simulink model "IEEE9_case"  (R2024b)
settings: Solver=FixedStepAuto  StartTime=0  StopTime=5  FixedStep=1e-7  RelTol=1e-3
values from neighbouring files (symbols this model uses):
  SG_D_1_D = 0.01056    [IEEE9_case_parameters.m]    (also in case1_parameters.m; case2_parameters.m; case3_parameters.m; case4_parameters.m)
  SG_D_1_EnableSaturation = 0    [IEEE9_case_parameters.m]    (also in case1_parameters.m; case2_parameters.m; case3_parameters.m; case4_parameters.m)
  SG_D_1_f0 = 60    [IEEE9_case_parameters.m]    (also in case1_parameters.m; case2_parameters.m; case3_parameters.m; case4_parameters.m)
  SG_D_1_H = 7.5    [IEEE9_case_parameters.m]    (also in case1_parameters.m; case2_parameters.m; case3_parameters.m; case4_parameters.m)
  SG_D_1_K_A = 20    [IEEE9_case_parameters.m]    (also in case1_parameters.m; case2_parameters.m; case3_parameters.m; case4_parameters.m)
  SG_D_1_K_E = 1.000000e+1    (= 10)    [IEEE9_case_parameters.m]    (also in case1_parameters.m; case2_parameters.m; case3_parameters.m; case4_parameters.m)
  SG_D_1_K_F = 2.363    [IEEE9_case_parameters.m]    (also in case1_parameters.m; case2_parameters.m; case3_parameters.m; case4_parameters.m)
  SG_D_1_K_s = 0.5    [IEEE9_case_parameters.m]    (also in case1_parameters.m = 5; case2_parameters.m = 5; case3_parameters.m = 5; case4_parameters.m = 5)
  SG_D_1_R_a = 0.001088    [IEEE9_case_parameters.m]    (also in case1_parameters.m; case2_parameters.m; case3_parameters.m; case4_parameters.m)
  SG_D_1_S_A = 1    [IEEE9_case_parameters.m]    (also in case1_parameters.m; case2_parameters.m; case3_parameters.m; case4_parameters.m)
  SG_D_1_S_B = 0.103    [IEEE9_case_parameters.m]    (also in case1_parameters.m; case2_parameters.m; case3_parameters.m; case4_parameters.m)
  SG_D_1_S_N = 10.659857    [IEEE9_case_parameters.m]    (also in case1_parameters.m; case2_parameters.m; case3_parameters.m; case4_parameters.m)
  SG_D_1_SpeedPara = 200    [IEEE9_case_parameters.m]    (also in case1_parameters.m; case2_parameters.m; case3_parameters.m; case4_parameters.m)
  SG_D_1_T_0 = 0.720173    [IEEE9_case_parameters.m]    (also in case1_parameters.m = 0.755522; case2_parameters.m = 0.808931; case3_parameters.m = 0.869402; case4_parameters.m = 0.729316)
  SG_D_1_T_1 = 0.3    [IEEE9_case_parameters.m]    (also in case1_parameters.m; case2_parameters.m; case3_parameters.m; case4_parameters.m)
  SG_D_1_T_2 = 0.05    [IEEE9_case_parameters.m]    (also in case1_parameters.m; case2_parameters.m; case3_parameters.m; case4_parameters.m)
  SG_D_1_T_3 = 0.02    [IEEE9_case_parameters.m]    (also in case1_parameters.m; case2_parameters.m; case3_parameters.m; case4_parameters.m)
  SG_D_1_T_4 = 0.005    [IEEE9_case_parameters.m]    (also in case1_parameters.m; case2_parameters.m; case3_parameters.m; case4_parameters.m)
  SG_D_1_T_A = 0.02    [IEEE9_case_parameters.m]    (also in case1_parameters.m; case2_parameters.m; case3_parameters.m; case4_parameters.m)
  SG_D_1_T_dd = 8.000000e+0    (= 8)    [IEEE9_case_parameters.m]    (also in case1_parameters.m; case2_parameters.m; case3_parameters.m; case4_parameters.m)
  SG_D_1_T_ddd = 0.04    [IEEE9_case_parameters.m]    (also in case1_parameters.m; case2_parameters.m; case3_parameters.m; case4_parameters.m)
  SG_D_1_T_E = 0.314    [IEEE9_case_parameters.m]    (also in case1_parameters.m; case2_parameters.m; case3_parameters.m; case4_parameters.m)
  SG_D_1_T_F = 0.35    [IEEE9_case_parameters.m]    (also in case1_parameters.m; case2_parameters.m; case3_parameters.m; case4_parameters.m)
  SG_D_1_T_qd = 0.8    [IEEE9_case_parameters.m]    (also in case1_parameters.m; case2_parameters.m; case3_parameters.m; case4_parameters.m)
  SG_D_1_T_qdd = 0.02    [IEEE9_case_parameters.m]    (also in case1_parameters.m; case2_parameters.m; case3_parameters.m; case4_parameters.m)
  SG_D_1_T_speed = 0.1    [IEEE9_case_parameters.m]    (also in case1_parameters.m = 200; case2_parameters.m = 200; case3_parameters.m = 200; case4_parameters.m = 200)
  SG_D_1_T_w = 0.5    [IEEE9_case_parameters.m]    (also in case1_parameters.m; case2_parameters.m; case3_parameters.m; case4_parameters.m)
  SG_D_1_V_ref = 1.990276    [IEEE9_case_parameters.m]    (also in case1_parameters.m = 2.042296; case2_parameters.m = 2.051388; case3_parameters.m = 2.089584; case4_parameters.m = 2.01845)
  SG_D_1_w_ref = 376.991118    [IEEE9_case_parameters.m]    (also in case1_parameters.m; case2_parameters.m; case3_parameters.m; case4_parameters.m)
  SG_D_1_wb = 6.000000e+1    (= 60)    [IEEE9_case_parameters.m]    (also in case1_parameters.m; case2_parameters.m; case3_parameters.m; case4_parameters.m)
  SG_D_1_x_d = 1.9    [IEEE9_case_parameters.m]    (also in case1_parameters.m; case2_parameters.m; case3_parameters.m; case4_parameters.m)
  SG_D_1_x_dd = 0.302    [IEEE9_case_parameters.m]    (also in case1_parameters.m; case2_parameters.m; case3_parameters.m; case4_parameters.m)
  SG_D_1_x_ddd = 0.204    [IEEE9_case_parameters.m]    (also in case1_parameters.m; case2_parameters.m; case3_parameters.m; case4_parameters.m)
  SG_D_1_x_l = 0.05    [IEEE9_case_parameters.m]    (also in case1_parameters.m; case2_parameters.m; case3_parameters.m; case4_parameters.m)
  SG_D_1_x_q = 1.3    [IEEE9_case_parameters.m]    (also in case1_parameters.m; case2_parameters.m; case3_parameters.m; case4_parameters.m)
  SG_D_1_x_qd = 0.5    [IEEE9_case_parameters.m]    (also in case1_parameters.m; case2_parameters.m; case3_parameters.m; case4_parameters.m)
  SG_D_1_x_qdd = 0.3    [IEEE9_case_parameters.m]    (also in case1_parameters.m; case2_parameters.m; case3_parameters.m; case4_parameters.m)
  SG_D_2_D = 0.02    [IEEE9_case_parameters.m]    (also in case1_parameters.m; case2_parameters.m; case3_parameters.m; case4_parameters.m)
  SG_D_2_EnableSaturation = 0    [IEEE9_case_parameters.m]    (also in case1_parameters.m; case2_parameters.m; case3_parameters.m; case4_parameters.m)
  SG_D_2_f0 = 60    [IEEE9_case_parameters.m]    (also in case1_parameters.m; case2_parameters.m; case3_parameters.m; case4_parameters.m)
  SG_D_2_H = 8.000000e+0    (= 8)    [IEEE9_case_parameters.m]    (also in case1_parameters.m; case2_parameters.m; case3_parameters.m; case4_parameters.m)
  SG_D_2_K_A = 20    [IEEE9_case_parameters.m]    (also in case1_parameters.m; case2_parameters.m; case3_parameters.m; case4_parameters.m)
  SG_D_2_K_E = 1.000000e+1    (= 10)    [IEEE9_case_parameters.m]    (also in case1_parameters.m; case2_parameters.m; case3_parameters.m; case4_parameters.m)
  SG_D_2_K_F = 2.363    [IEEE9_case_parameters.m]    (also in case1_parameters.m; case2_parameters.m; case3_parameters.m; case4_parameters.m)
  SG_D_2_K_s = 0.5    [IEEE9_case_parameters.m]    (also in case1_parameters.m = 4; case2_parameters.m = 4; case3_parameters.m = 4; case4_parameters.m = 4)
  SG_D_2_R_a = 0.001088    [IEEE9_case_parameters.m]    (also in case1_parameters.m; case2_parameters.m; case3_parameters.m; case4_parameters.m)
  SG_D_2_S_A = 1    [IEEE9_case_parameters.m]    (also in case1_parameters.m; case2_parameters.m; case3_parameters.m; case4_parameters.m)
  SG_D_2_S_B = 0.103    [IEEE9_case_parameters.m]    (also in case1_parameters.m; case2_parameters.m; case3_parameters.m; case4_parameters.m)
  SG_D_2_S_N = 10.659857    [IEEE9_case_parameters.m]    (also in case1_parameters.m; case2_parameters.m; case3_parameters.m; case4_parameters.m)
  SG_D_2_SpeedPara = 200    [IEEE9_case_parameters.m]    (also in case1_parameters.m; case2_parameters.m; case3_parameters.m; case4_parameters.m)
  SG_D_2_T_0 = 1.632913    [IEEE9_case_parameters.m]    (also in case1_parameters.m = 1.632925; case2_parameters.m = 1.632915; case3_parameters.m = 1.632914; case4_parameters.m = 1.632927)
  SG_D_2_T_1 = 0.2    [IEEE9_case_parameters.m]    (also in case1_parameters.m; case2_parameters.m; case3_parameters.m; case4_parameters.m)
  SG_D_2_T_2 = 0.05    [IEEE9_case_parameters.m]    (also in case1_parameters.m; case2_parameters.m; case3_parameters.m; case4_parameters.m)
  SG_D_2_T_3 = 0.02    [IEEE9_case_parameters.m]    (also in case1_parameters.m; case2_parameters.m; case3_parameters.m; case4_parameters.m)
  SG_D_2_T_4 = 0.005    [IEEE9_case_parameters.m]    (also in case1_parameters.m; case2_parameters.m; case3_parameters.m; case4_parameters.m)
  SG_D_2_T_A = 0.02    [IEEE9_case_parameters.m]    (also in case1_parameters.m; case2_parameters.m; case3_parameters.m; case4_parameters.m)
  SG_D_2_T_dd = 7.9    [IEEE9_case_parameters.m]    (also in case1_parameters.m; case2_parameters.m; case3_parameters.m; case4_parameters.m)
  SG_D_2_T_ddd = 0.04    [IEEE9_case_parameters.m]    (also in case1_parameters.m; case2_parameters.m; case3_parameters.m; case4_parameters.m)
  SG_D_2_T_E = 0.314    [IEEE9_case_parameters.m]    (also in case1_parameters.m; case2_parameters.m; case3_parameters.m; case4_parameters.m)
  SG_D_2_T_F = 0.35    [IEEE9_case_parameters.m]    (also in case1_parameters.m; case2_parameters.m; case3_parameters.m; case4_parameters.m)
  SG_D_2_T_qd = 0.8    [IEEE9_case_parameters.m]    (also in case1_parameters.m; case2_parameters.m; case3_parameters.m; case4_parameters.m)
  SG_D_2_T_qdd = 0.015    [IEEE9_case_parameters.m]    (also in case1_parameters.m; case2_parameters.m; case3_parameters.m; case4_parameters.m)
  SG_D_2_T_speed = 0.1    [IEEE9_case_parameters.m]    (also in case1_parameters.m = 150; case2_parameters.m = 150; case3_parameters.m = 150; case4_parameters.m = 150)
  SG_D_2_T_w = 0.35    [IEEE9_case_parameters.m]    (also in case1_parameters.m; case2_parameters.m; case3_parameters.m; case4_parameters.m)
  SG_D_2_V_ref = 2.58547    [IEEE9_case_parameters.m]    (also in case1_parameters.m = 2.597896; case2_parameters.m = 2.587136; case3_parameters.m = 2.586042; case4_parameters.m = 2.599679)
  SG_D_2_w_ref = 376.991118    [IEEE9_case_parameters.m]    (also in case1_parameters.m; case2_parameters.m; case3_parameters.m; case4_parameters.m)
  SG_D_2_wb = 6.000000e+1    (= 60)    [IEEE9_case_parameters.m]    (also in case1_parameters.m; case2_parameters.m; case3_parameters.m; case4_parameters.m)
  SG_D_2_x_d = 1.8    [IEEE9_case_parameters.m]    (also in case1_parameters.m; case2_parameters.m; case3_parameters.m; case4_parameters.m)
  SG_D_2_x_dd = 0.302    [IEEE9_case_parameters.m]    (also in case1_parameters.m; case2_parameters.m; case3_parameters.m; case4_parameters.m)
  SG_D_2_x_ddd = 0.204    [IEEE9_case_parameters.m]    (also in case1_parameters.m; case2_parameters.m; case3_parameters.m; case4_parameters.m)
  SG_D_2_x_l = 0.05    [IEEE9_case_parameters.m]    (also in case1_parameters.m; case2_parameters.m; case3_parameters.m; case4_parameters.m)
  SG_D_2_x_q = 1.25    [IEEE9_case_parameters.m]    (also in case1_parameters.m; case2_parameters.m; case3_parameters.m; case4_parameters.m)
  SG_D_2_x_qd = 0.5    [IEEE9_case_parameters.m]    (also in case1_parameters.m; case2_parameters.m; case3_parameters.m; case4_parameters.m)
  SG_D_2_x_qdd = 0.3    [IEEE9_case_parameters.m]    (also in case1_parameters.m; case2_parameters.m; case3_parameters.m; case4_parameters.m)
  SG_D_3_D = 0.02    [IEEE9_case_parameters.m]    (also in case1_parameters.m; case2_parameters.m; case3_parameters.m; case4_parameters.m)
  SG_D_3_EnableSaturation = 0    [IEEE9_case_parameters.m]    (also in case1_parameters.m; case2_parameters.m; case3_parameters.m; case4_parameters.m)
  SG_D_3_f0 = 60    [IEEE9_case_parameters.m]    (also in case1_parameters.m; case2_parameters.m; case3_parameters.m; case4_parameters.m)
  SG_D_3_H = 7.7    [IEEE9_case_parameters.m]    (also in case1_parameters.m; case2_parameters.m; case3_parameters.m; case4_parameters.m)
  SG_D_3_K_A = 20    [IEEE9_case_parameters.m]    (also in case1_parameters.m; case2_parameters.m; case3_parameters.m; case4_parameters.m)
  SG_D_3_K_E = 1.000000e+1    (= 10)    [IEEE9_case_parameters.m]    (also in case1_parameters.m; case2_parameters.m; case3_parameters.m; case4_parameters.m)
  SG_D_3_K_F = 2.363    [IEEE9_case_parameters.m]    (also in case1_parameters.m; case2_parameters.m; case3_parameters.m; case4_parameters.m)
  SG_D_3_K_s = 0.2    [IEEE9_case_parameters.m]    (also in case1_parameters.m = 2; case2_parameters.m = 2; case3_parameters.m = 2; case4_parameters.m = 2)
  SG_D_3_R_a = 0.001088    [IEEE9_case_parameters.m]    (also in case1_parameters.m; case2_parameters.m; case3_parameters.m; case4_parameters.m)
  SG_D_3_S_A = 1    [IEEE9_case_parameters.m]    (also in case1_parameters.m; case2_parameters.m; case3_parameters.m; case4_parameters.m)
  SG_D_3_S_B = 0.103    [IEEE9_case_parameters.m]    (also in case1_parameters.m; case2_parameters.m; case3_parameters.m; case4_parameters.m)
  SG_D_3_S_N = 10.659857    [IEEE9_case_parameters.m]    (also in case1_parameters.m; case2_parameters.m; case3_parameters.m; case4_parameters.m)
  SG_D_3_SpeedPara = 200    [IEEE9_case_parameters.m]    (also in case1_parameters.m; case2_parameters.m; case3_parameters.m; case4_parameters.m)
  SG_D_3_T_0 = 0.850788    [IEEE9_case_parameters.m]    (also in case1_parameters.m = 0.850786; case2_parameters.m = 0.850787; case3_parameters.m; case4_parameters.m = 0.850786)
  SG_D_3_T_1 = 0.2    [IEEE9_case_parameters.m]    (also in case1_parameters.m; case2_parameters.m; case3_parameters.m; case4_parameters.m)
  SG_D_3_T_2 = 0.05    [IEEE9_case_parameters.m]    (also in case1_parameters.m; case2_parameters.m; case3_parameters.m; case4_parameters.m)
  SG_D_3_T_3 = 0.02    [IEEE9_case_parameters.m]    (also in case1_parameters.m; case2_parameters.m; case3_parameters.m; case4_parameters.m)
  SG_D_3_T_4 = 0.005    [IEEE9_case_parameters.m]    (also in case1_parameters.m; case2_parameters.m; case3_parameters.m; case4_parameters.m)
  SG_D_3_T_A = 0.02    [IEEE9_case_parameters.m]    (also in case1_parameters.m; case2_parameters.m; case3_parameters.m; case4_parameters.m)
  SG_D_3_T_dd = 8.1    [IEEE9_case_parameters.m]    (also in case1_parameters.m; case2_parameters.m; case3_parameters.m; case4_parameters.m)
  SG_D_3_T_ddd = 0.04    [IEEE9_case_parameters.m]    (also in case1_parameters.m; case2_parameters.m; case3_parameters.m; case4_parameters.m)
  SG_D_3_T_E = 0.314    [IEEE9_case_parameters.m]    (also in case1_parameters.m; case2_parameters.m; case3_parameters.m; case4_parameters.m)
  SG_D_3_T_F = 0.35    [IEEE9_case_parameters.m]    (also in case1_parameters.m; case2_parameters.m; case3_parameters.m; case4_parameters.m)
  SG_D_3_T_qd = 0.8    [IEEE9_case_parameters.m]    (also in case1_parameters.m; case2_parameters.m; case3_parameters.m; case4_parameters.m)
  SG_D_3_T_qdd = 0.015    [IEEE9_case_parameters.m]    (also in case1_parameters.m; case2_parameters.m; case3_parameters.m; case4_parameters.m)
  SG_D_3_T_speed = 0.1    [IEEE9_case_parameters.m]    (also in case1_parameters.m = 180; case2_parameters.m = 180; case3_parameters.m = 180; case4_parameters.m = 180)
  SG_D_3_T_w = 0.4    [IEEE9_case_parameters.m]    (also in case1_parameters.m; case2_parameters.m; case3_parameters.m; case4_parameters.m)
  SG_D_3_V_ref = 1.892727    [IEEE9_case_parameters.m]    (also in case1_parameters.m = 1.906439; case2_parameters.m = 1.895535; case3_parameters.m = 1.892105; case4_parameters.m = 1.906598)
  SG_D_3_w_ref = 376.991118    [IEEE9_case_parameters.m]    (also in case1_parameters.m; case2_parameters.m; case3_parameters.m; case4_parameters.m)
  SG_D_3_wb = 6.000000e+1    (= 60)    [IEEE9_case_parameters.m]    (also in case1_parameters.m; case2_parameters.m; case3_parameters.m; case4_parameters.m)
  SG_D_3_x_d = 1.85    [IEEE9_case_parameters.m]    (also in case1_parameters.m; case2_parameters.m; case3_parameters.m; case4_parameters.m)
  SG_D_3_x_dd = 0.302    [IEEE9_case_parameters.m]    (also in case1_parameters.m; case2_parameters.m; case3_parameters.m; case4_parameters.m)
  SG_D_3_x_ddd = 0.204    [IEEE9_case_parameters.m]    (also in case1_parameters.m; case2_parameters.m; case3_parameters.m; case4_parameters.m)
  SG_D_3_x_l = 0.05    [IEEE9_case_parameters.m]    (also in case1_parameters.m; case2_parameters.m; case3_parameters.m; case4_parameters.m)
  SG_D_3_x_q = 1.2    [IEEE9_case_parameters.m]    (also in case1_parameters.m; case2_parameters.m; case3_parameters.m; case4_parameters.m)
  SG_D_3_x_qd = 0.5    [IEEE9_case_parameters.m]    (also in case1_parameters.m; case2_parameters.m; case3_parameters.m; case4_parameters.m)
  SG_D_3_x_qdd = 0.3    [IEEE9_case_parameters.m]    (also in case1_parameters.m; case2_parameters.m; case3_parameters.m; case4_parameters.m)
(part 7 of 12)

== system IEEE9_case/SG_D_1/i_q_SG_D_1_block ==
  note: i_q_SG_D_1 in IEEE9_case
      | $-\frac{\sin\left(\theta _{\mathrm{SG},D,1}\right)\,\left(\psi _{q,\mathrm{SG},D,1}+\frac{\psi _{\mathrm{gq},\mathrm{SG},D,1}\,\left(x_{l}-x_{\mathrm{qdd}}\right)}{x_{l}-x_{\mathrm{qd}}}+\frac{\psi _{\mathrm{kq},\mathrm{SG},D,1}\,\left(x_{\mathrm{qd}}-x_{\mathrm{qdd}}\right)}{x_{l}-x_{\mathrm{qd}}}\right)}{x_{\mathrm{qdd}}}-\frac{\cos\left(\theta _{\mathrm{SG},D,1}\right)\,\left(\frac{\psi _{\mathrm{1d},\mathrm{SG},D,1}\,\left(x_{\mathrm{dd}}-x_{\mathrm{ddd}}\right)}{x_{\mathrm{dd}}-x_{l}}-\psi _{d,\mathrm{SG},D,1}+\frac{\psi _{\mathrm{fd},\mathrm{SG},D,1}\,\left(x_{\mathrm{ddd}}-x_{l}\right)}{x_{\mathrm{dd}}-x_{l}}\right)}{x_{\mathrm{ddd}}}$
      | Automatically generated on 2025-11-01 08:48:16 .
  State_psi_gq_SG_D_1_b3414 : Inport
  State_psi_kq_SG_D_1_642ee : Inport  Port=2
  State_psi_q_SG_D_1_76ae1 : Inport  Port=3
  State_theta_SG_D_1_7319b : Inport  Port=4
  State_psi_1d_SG_D_1_b02a1 : Inport  Port=5
  State_psi_d_SG_D_1_d4abd : Inport  Port=6
  State_psi_fd_SG_D_1_7b602 : Inport  Port=7
  State_theta_SG_D_1_dd7cd : Inport  Port=8
  Add_1276b : Sum
  Add_4f3d3 : Sum
  Add_5fd68 : Sum
  Add_682ce : Sum
  Add_9f7ef : Sum
  Add_a5d11 : Sum
  Constant_-1_237cd : Constant  Value=-1
  Constant_-1_6e66d : Constant  Value=-1
  Constant_-1_863bd : Constant  Value=-1
  Constant_-1_a124f : Constant  Value=-1
  Constant_-1_b4d74 : Constant  Value=-1
  Constant_x_dd_114fa : Constant  Value=x_dd
  Constant_x_dd_1296b : Constant  Value=x_dd
  Constant_x_dd_c876c : Constant  Value=x_dd
  Constant_x_ddd_14b41 : Constant  Value=x_ddd
  Constant_x_ddd_ff12c : Constant  Value=x_ddd
  Constant_x_ddd_ff2d6 : Constant  Value=x_ddd
  Constant_x_l_1cade : Constant  Value=x_l
  Constant_x_l_483a3 : Constant  Value=x_l
  Constant_x_l_64d13 : Constant  Value=x_l
  Constant_x_l_a4e1e : Constant  Value=x_l
  Constant_x_l_cd8ca : Constant  Value=x_l
  Constant_x_l_d0656 : Constant  Value=x_l
  Constant_x_qd_1d796 : Constant  Value=x_qd
  Constant_x_qd_83eee : Constant  Value=x_qd
  Constant_x_qd_e34c4 : Constant  Value=x_qd
  Constant_x_qdd_61e6e : Constant  Value=x_qdd
  Constant_x_qdd_66c35 : Constant  Value=x_qdd
  Constant_x_qdd_dfec3 : Constant  Value=x_qdd
  Divide_1c872 : Product  Inputs=*/
  Divide_38445 : Product  Inputs=*/
  Divide_64305 : Product  Inputs=*/
  Divide_7e9bc : Product  Inputs=*/
  Divide_96a6f : Product  Inputs=*/
  Divide_c0a1a : Product  Inputs=*/
  MathFunc_cos_86739 : Trigonometry  Operator=cos
  MathFunc_sin_e52d9 : Trigonometry
  Product_01f65 : Product
  Product_26f15 : Product
  Product_29f51 : Product
  Product_30034 : Product
  Product_969d5 : Product
  Product_a1107 : Product
  Product_ba82a : Product
  Product_cc270 : Product
  Product_d51fe : Product
  Product_e3a3e : Product
  Product_ee1a4 : Product
  Subtract_4f1c6 : Sum  Inputs=+-
  Subtract_7397b : Sum  Inputs=+-
  Subtract_c436c : Sum  Inputs=+-
  Subtract_c5ad8 : Sum  Inputs=+-
  Subtract_d75bc : Sum  Inputs=+-
  Subtract_e4c24 : Sum  Inputs=+-
  Subtract_fb039 : Sum  Inputs=+-
  Blockout_i_q_SG_D_1_db7dd : Outport
  wires:
  State_theta_SG_D_1_dd7cd/1 -> MathFunc_cos_86739/1
  State_psi_fd_SG_D_1_7b602/1 -> Product_01f65/1
  Constant_-1_863bd/1 -> Product_ba82a/1
  Constant_x_l_a4e1e/1 -> Product_ba82a/2
  Subtract_7397b/1 -> Product_01f65/2
  Constant_x_l_483a3/1 -> Subtract_d75bc/2
  Product_ba82a/1 -> Add_1276b/1
  Constant_x_qdd_66c35/1 -> Add_1276b/2
  Constant_x_qd_1d796/1 -> Subtract_c5ad8/1
  Constant_x_qdd_61e6e/1 -> Divide_96a6f/2
  MathFunc_sin_e52d9/1 -> Product_26f15/2
  Constant_-1_b4d74/1 -> Product_29f51/1
  Constant_x_qdd_dfec3/1 -> Subtract_c5ad8/2
  Add_a5d11/1 -> Product_ee1a4/2
  Product_30034/1 -> Divide_38445/1
  Constant_x_l_cd8ca/1 -> Product_29f51/2
  Constant_-1_a124f/1 -> Product_d51fe/1
  Constant_x_l_64d13/1 -> Product_d51fe/2
  State_psi_gq_SG_D_1_b3414/1 -> Product_30034/1
  Add_1276b/1 -> Product_30034/2
  Divide_7e9bc/1 -> Add_9f7ef/1
  Product_29f51/1 -> Add_4f3d3/1
  Divide_96a6f/1 -> Add_5fd68/1
  Constant_x_qd_83eee/1 -> Add_4f3d3/2
  State_psi_kq_SG_D_1_642ee/1 -> Product_a1107/1
  Add_9f7ef/1 -> Subtract_e4c24/1
  Subtract_c5ad8/1 -> Product_a1107/2
  Divide_38445/1 -> Subtract_4f1c6/1
  Add_4f3d3/1 -> Divide_38445/2
  Product_d51fe/1 -> Add_682ce/1
  Constant_x_qd_e34c4/1 -> Add_682ce/2
  Constant_-1_6e66d/1 -> Product_cc270/1
  MathFunc_cos_86739/1 -> Product_969d5/2
  Product_01f65/1 -> Divide_64305/1
  State_psi_1d_SG_D_1_b02a1/1 -> Product_cc270/2
  Constant_x_l_d0656/1 -> Subtract_c436c/2
  Constant_x_dd_1296b/1 -> Subtract_fb039/1
  Divide_64305/1 -> Subtract_e4c24/2
  Constant_x_ddd_ff2d6/1 -> Subtract_fb039/2
  Product_969d5/1 -> Divide_1c872/1
  Product_a1107/1 -> Divide_c0a1a/1
  Product_cc270/1 -> Product_e3a3e/1
  Add_682ce/1 -> Divide_c0a1a/2
  Subtract_fb039/1 -> Product_e3a3e/2
  State_psi_d_SG_D_1_d4abd/1 -> Add_9f7ef/2
  Constant_x_dd_c876c/1 -> Subtract_d75bc/1
  Constant_x_ddd_ff12c/1 -> Subtract_7397b/1
  Constant_x_l_1cade/1 -> Subtract_7397b/2
  Divide_1c872/1 -> Add_5fd68/2
  Divide_c0a1a/1 -> Subtract_4f1c6/2
  State_theta_SG_D_1_7319b/1 -> MathFunc_sin_e52d9/1
  Product_e3a3e/1 -> Divide_7e9bc/1
  Subtract_d75bc/1 -> Divide_7e9bc/2
  Constant_x_dd_114fa/1 -> Subtract_c436c/1
  Subtract_4f1c6/1 -> Add_a5d11/1
  State_psi_q_SG_D_1_76ae1/1 -> Add_a5d11/2
  Subtract_c436c/1 -> Divide_64305/2
  Subtract_e4c24/1 -> Product_969d5/1
  Constant_-1_237cd/1 -> Product_ee1a4/1
  Product_ee1a4/1 -> Product_26f15/1
  Product_26f15/1 -> Divide_96a6f/1
  Constant_x_ddd_14b41/1 -> Divide_1c872/2
  Add_5fd68/1 -> Blockout_i_q_SG_D_1_db7dd/1

== system IEEE9_case/SG_D_1/theta_SG_D_1_out_block ==
  note: theta_SG_D_1_out in IEEE9_case
      | $\theta _{\mathrm{SG},D,1}$
      | Automatically generated on 2025-11-01 08:48:21 .
  State_theta_SG_D_1_a22d0 : Inport
  Blockout_theta_SG_D_1_out_f2916 : Outport
  wires:
  State_theta_SG_D_1_a22d0/1 -> Blockout_theta_SG_D_1_out_f2916/1

== system IEEE9_case/SG_D_1/w_SG_D_1_out_block ==
  note: w_SG_D_1_out in IEEE9_case
      | $w_{\mathrm{SG},D,1}$
      | Automatically generated on 2025-11-01 08:48:21 .
  State_w_SG_D_1_9aa86 : Inport
  Blockout_w_SG_D_1_out_73f9d : Outport
  wires:
  State_w_SG_D_1_9aa86/1 -> Blockout_w_SG_D_1_out_73f9d/1

== system IEEE9_case/SG_D_2/T_e_SG_D_2_block ==
  note: T_e_SG_D_2 in IEEE9_case
      | $-\frac{\psi _{d,\mathrm{SG},D,2}\,\left(\psi _{q,\mathrm{SG},D,2}+\frac{\psi _{\mathrm{gq},\mathrm{SG},D,2}\,\left(x_{l}-x_{\mathrm{qdd}}\right)}{x_{l}-x_{\mathrm{qd}}}+\frac{\psi _{\mathrm{kq},\mathrm{SG},D,2}\,\left(x_{\mathrm{qd}}-x_{\mathrm{qdd}}\right)}{x_{l}-x_{\mathrm{qd}}}\right)}{x_{\mathrm{qdd}}}-\frac{\psi _{q,\mathrm{SG},D,2}\,\left(\frac{\psi _{\mathrm{1d},\mathrm{SG},D,2}\,\left(x_{\mathrm{dd}}-x_{\mathrm{ddd}}\right)}{x_{\mathrm{dd}}-x_{l}}-\psi _{d,\mathrm{SG},D,2}+\frac{\psi _{\mathrm{fd},\mathrm{SG},D,2}\,\left(x_{\mathrm{ddd}}-x_{l}\right)}{x_{\mathrm{dd}}-x_{l}}\right)}{x_{\mathrm{ddd}}}$
      | Automatically generated on 2025-11-01 08:49:28 .
  State_psi_d_SG_D_2_ab5a2 : Inport
  State_psi_gq_SG_D_2_748c1 : Inport  Port=2
  State_psi_kq_SG_D_2_3e69f : Inport  Port=3
  State_psi_q_SG_D_2_b203e : Inport  Port=4
  State_psi_q_SG_D_2_f483f : Inport  Port=5
  State_psi_1d_SG_D_2_95086 : Inport  Port=6
  State_psi_d_SG_D_2_9e58e : Inport  Port=7
  State_psi_fd_SG_D_2_499b8 : Inport  Port=8
  Add_1f388 : Sum
  Add_53f88 : Sum
  Add_58979 : Sum
  Add_5dfbe : Sum
  Add_ae658 : Sum
  Add_b1ae1 : Sum
  Constant_-1_19e25 : Constant  Value=-1
  Constant_-1_37556 : Constant  Value=-1
  Constant_-1_55c25 : Constant  Value=-1
  Constant_-1_c6ebe : Constant  Value=-1
  Constant_-1_d6559 : Constant  Value=-1
  Constant_x_dd_2ab23 : Constant  Value=x_dd
  Constant_x_dd_3d0c9 : Constant  Value=x_dd
  Constant_x_dd_fc5a4 : Constant  Value=x_dd
  Constant_x_ddd_119f4 : Constant  Value=x_ddd
  Constant_x_ddd_745ee : Constant  Value=x_ddd
  Constant_x_ddd_ee87d : Constant  Value=x_ddd
  Constant_x_l_15e6c : Constant  Value=x_l
  Constant_x_l_1b750 : Constant  Value=x_l
  Constant_x_l_62c33 : Constant  Value=x_l
  Constant_x_l_75781 : Constant  Value=x_l
  Constant_x_l_77dcb : Constant  Value=x_l
  Constant_x_l_82014 : Constant  Value=x_l
  Constant_x_qd_9d2e7 : Constant  Value=x_qd
  Constant_x_qd_aa90c : Constant  Value=x_qd
  Constant_x_qd_c48b2 : Constant  Value=x_qd
  Constant_x_qdd_56e24 : Constant  Value=x_qdd
  Constant_x_qdd_d545b : Constant  Value=x_qdd
  Constant_x_qdd_f204c : Constant  Value=x_qdd
  Divide_77255 : Product  Inputs=*/
  Divide_bbde5 : Product  Inputs=*/
  Divide_c00c4 : Product  Inputs=*/
  Divide_cd7d4 : Product  Inputs=*/
  Divide_f8c6c : Product  Inputs=*/
  Divide_fd8ad : Product  Inputs=*/
  Product_19829 : Product
  Product_1b6fa : Product
  Product_4b4ab : Product
  Product_52bf8 : Product
  Product_59e04 : Product
  Product_74056 : Product
  Product_9308c : Product
  Product_93fd4 : Product
  Product_a5460 : Product
  Product_b03b7 : Product
  Product_c0f36 : Product
  Subtract_18d7b : Sum  Inputs=+-
  Subtract_49c75 : Sum  Inputs=+-
  Subtract_4eb9c : Sum  Inputs=+-
  Subtract_8449f : Sum  Inputs=+-
  Subtract_9b2c1 : Sum  Inputs=+-
  Subtract_b4907 : Sum  Inputs=+-
  Subtract_deee9 : Sum  Inputs=+-
  Blockout_T_e_SG_D_2_66ce8 : Outport
  wires:
  Constant_-1_37556/1 -> Product_93fd4/1
  Divide_c00c4/1 -> Subtract_8449f/1
  Constant_-1_19e25/1 -> Product_74056/1
  Constant_x_l_1b750/1 -> Product_74056/2
  Constant_x_qd_c48b2/1 -> Subtract_4eb9c/1
  Product_9308c/1 -> Divide_c00c4/1
  Product_74056/1 -> Add_53f88/1
  Divide_fd8ad/1 -> Subtract_deee9/2
  Constant_x_qdd_f204c/1 -> Subtract_4eb9c/2
  Constant_x_qdd_56e24/1 -> Divide_bbde5/2
  Constant_x_ddd_119f4/1 -> Subtract_18d7b/2
  Constant_x_qdd_d545b/1 -> Add_53f88/2
  Constant_x_l_77dcb/1 -> Product_93fd4/2
  Constant_-1_d6559/1 -> Product_19829/1
  Constant_x_l_75781/1 -> Product_19829/2
  Constant_-1_55c25/1 -> Product_1b6fa/1
  State_psi_1d_SG_D_2_95086/1 -> Product_1b6fa/2
  Constant_x_dd_3d0c9/1 -> Subtract_18d7b/1
  Divide_cd7d4/1 -> Subtract_8449f/2
  State_psi_gq_SG_D_2_748c1/1 -> Product_9308c/1
  Add_53f88/1 -> Product_9308c/2
  Subtract_8449f/1 -> Add_5dfbe/1
  Constant_x_dd_fc5a4/1 -> Subtract_b4907/1
  Product_93fd4/1 -> Add_b1ae1/1
  Product_a5460/1 -> Product_4b4ab/1
  Constant_x_qd_aa90c/1 -> Add_b1ae1/2
  State_psi_kq_SG_D_2_3e69f/1 -> Product_b03b7/1
  Subtract_4eb9c/1 -> Product_b03b7/2
  Product_19829/1 -> Add_1f388/1
  State_psi_q_SG_D_2_f483f/1 -> Product_52bf8/1
  Constant_x_qd_9d2e7/1 -> Add_1f388/2
  Product_1b6fa/1 -> Product_59e04/1
  Divide_77255/1 -> Add_58979/2
  Subtract_18d7b/1 -> Product_59e04/2
  Constant_x_l_82014/1 -> Subtract_b4907/2
  Constant_x_ddd_ee87d/1 -> Subtract_49c75/1
  Constant_x_dd_2ab23/1 -> Subtract_9b2c1/1
  Constant_x_l_15e6c/1 -> Subtract_49c75/2
  Add_58979/1 -> Blockout_T_e_SG_D_2_66ce8/1
  Add_b1ae1/1 -> Divide_c00c4/2
  Product_b03b7/1 -> Divide_cd7d4/1
  Product_4b4ab/1 -> Divide_bbde5/1
  State_psi_d_SG_D_2_ab5a2/1 -> Product_a5460/2
  Add_1f388/1 -> Divide_cd7d4/2
  Product_59e04/1 -> Divide_f8c6c/1
  Subtract_b4907/1 -> Divide_f8c6c/2
  Constant_x_l_62c33/1 -> Subtract_9b2c1/2
  State_psi_fd_SG_D_2_499b8/1 -> Product_c0f36/1
  Constant_x_ddd_745ee/1 -> Divide_77255/2
  Product_52bf8/1 -> Divide_77255/1
  Subtract_49c75/1 -> Product_c0f36/2
  Divide_f8c6c/1 -> Add_ae658/1
  State_psi_d_SG_D_2_9e58e/1 -> Add_ae658/2
  Add_ae658/1 -> Subtract_deee9/1
  Product_c0f36/1 -> Divide_fd8ad/1
  Subtract_9b2c1/1 -> Divide_fd8ad/2
  Constant_-1_c6ebe/1 -> Product_a5460/1
  State_psi_q_SG_D_2_b203e/1 -> Add_5dfbe/2
  Add_5dfbe/1 -> Product_4b4ab/2
  Subtract_deee9/1 -> Product_52bf8/2
  Divide_bbde5/1 -> Add_58979/1

== system IEEE9_case/SG_D_2/d_E_fd_SG_D_2_block ==
  note: d_E_fd_SG_D_2 in IEEE9_case
      | $\frac{V_{f,\mathrm{SG},D,2}-E_{\mathrm{fd},\mathrm{SG},D,2}\,K_{E}}{T_{E}}$
      | Automatically generated on 2025-11-01 08:49:11 .
  State_E_fd_SG_D_2_1a251 : Inport
  State_V_f_SG_D_2_a732e : Inport  Port=2
  Add_c15cb : Sum
  Constant_-1_f0724 : Constant  Value=-1
  Constant_K_E_4cfac : Constant  Value=K_E
  Constant_T_E_4e057 : Constant  Value=T_E
  Divide_f1acc : Product  Inputs=*/
  Product_67dc1 : Product
  Product_8dd90 : Product
  Blockout_d_E_fd_SG_D_2_9aa5a : Outport
  wires:
  Constant_-1_f0724/1 -> Product_8dd90/1
  State_E_fd_SG_D_2_1a251/1 -> Product_8dd90/2
  Product_8dd90/1 -> Product_67dc1/1
  Constant_K_E_4cfac/1 -> Product_67dc1/2
  Product_67dc1/1 -> Add_c15cb/1
  Constant_T_E_4e057/1 -> Divide_f1acc/2
  State_V_f_SG_D_2_a732e/1 -> Add_c15cb/2
  Add_c15cb/1 -> Divide_f1acc/1
  Divide_f1acc/1 -> Blockout_d_E_fd_SG_D_2_9aa5a/1

== system IEEE9_case/SG_D_2/d_Px_1_SG_D_2_block ==
  note: d_Px_1_SG_D_2 in IEEE9_case
      | $\frac{w_{\mathrm{SG},D,2}-2\,\pi \,f_{0}}{T_{w}}-\frac{\mathrm{Px}_{1,\mathrm{SG},D,2}}{T_{w}}$
      | Automatically generated on 2025-11-01 08:49:12 .
  State_Px_1_SG_D_2_4c7b1 : Inport
  State_w_SG_D_2_d8062 : Inport  Port=2
  Add_87559 : Sum
  Add_ecf39 : Sum
  Constant_-1_a7c9a : Constant  Value=-1
  Constant_-2.0_7e3ad : Constant  Value=-2.0
  Constant_T_w_bb843 : Constant  Value=T_w
  Constant_T_w_d675a : Constant  Value=T_w
  Constant_f0_00e9c : Constant  Value=f0
  Constant_pi_35444 : Constant  Value=pi
  Divide_22774 : Product  Inputs=*/
  Divide_351f9 : Product  Inputs=*/
  Product_0c290 : Product
  Product_2254f : Product
  Product_f99df : Product
  Blockout_d_Px_1_SG_D_2_5e8fa : Outport
  wires:
  Constant_-2.0_7e3ad/1 -> Product_2254f/1
  State_w_SG_D_2_d8062/1 -> Add_87559/2
  Constant_pi_35444/1 -> Product_2254f/2
  Product_2254f/1 -> Product_f99df/1
  Constant_f0_00e9c/1 -> Product_f99df/2
  Constant_-1_a7c9a/1 -> Product_0c290/1
  State_Px_1_SG_D_2_4c7b1/1 -> Product_0c290/2
  Product_f99df/1 -> Add_87559/1
  Product_0c290/1 -> Divide_351f9/1
  Constant_T_w_bb843/1 -> Divide_351f9/2
  Add_87559/1 -> Divide_22774/1
  Constant_T_w_d675a/1 -> Divide_22774/2
  Divide_351f9/1 -> Add_ecf39/1
  Divide_22774/1 -> Add_ecf39/2
  Add_ecf39/1 -> Blockout_d_Px_1_SG_D_2_5e8fa/1

== system IEEE9_case/SG_D_2/d_Px_2_SG_D_2_block ==
  note: d_Px_2_SG_D_2 in IEEE9_case
      | $\frac{\mathrm{Px}_{1,\mathrm{SG},D,2}-T_{2}\,\left(\frac{\mathrm{Px}_{1,\mathrm{SG},D,2}}{T_{w}}-\frac{w_{\mathrm{SG},D,2}-2\,\pi \,f_{0}}{T_{w}}\right)}{T_{1}}-\frac{\mathrm{Px}_{2,\mathrm{SG},D,2}}{T_{1}}$
      | Automatically generated on 2025-11-01 08:49:14 .
  State_Px_2_SG_D_2_06eab : Inport
  State_Px_1_SG_D_2_be7f9 : Inport  Port=2
  State_Px_1_SG_D_2_fde36 : Inport  Port=3
  State_w_SG_D_2_c021f : Inport  Port=4
  Add_05d88 : Sum
  Add_9667d : Sum
  Add_a5b72 : Sum
  Add_b38f2 : Sum
  Constant_-1_30d25 : Constant  Value=-1
  Constant_-1_eb528 : Constant  Value=-1
  Constant_-2.0_6b63d : Constant  Value=-2.0
  Constant_T_1_b6bc0 : Constant  Value=T_1
  Constant_T_1_fc97c : Constant  Value=T_1
  Constant_T_2_01690 : Constant  Value=T_2
  Constant_T_w_abd95 : Constant  Value=T_w
  Constant_T_w_e0452 : Constant  Value=T_w
  Constant_f0_c845d : Constant  Value=f0
  Constant_pi_8488f : Constant  Value=pi
  Divide_6c654 : Product  Inputs=*/
  Divide_83357 : Product  Inputs=*/
  Divide_96d2f : Product  Inputs=*/
  Divide_9cc5b : Product  Inputs=*/
  Product_7477e : Product
  Product_7b0e8 : Product
  Product_7c664 : Product
  Product_b2540 : Product
  Product_d1f4d : Product
  Blockout_d_Px_2_SG_D_2_a6ada : Outport
  wires:
  Constant_-1_30d25/1 -> Product_7b0e8/1
  Constant_-2.0_6b63d/1 -> Product_b2540/1
  Product_7477e/1 -> Add_05d88/2
  State_w_SG_D_2_c021f/1 -> Add_a5b72/2
  Constant_pi_8488f/1 -> Product_b2540/2
  Product_b2540/1 -> Product_d1f4d/1
  State_Px_1_SG_D_2_fde36/1 -> Product_7c664/2
  Constant_f0_c845d/1 -> Product_d1f4d/2
  State_Px_2_SG_D_2_06eab/1 -> Product_7b0e8/2
  Constant_-1_eb528/1 -> Product_7c664/1
  Product_d1f4d/1 -> Add_a5b72/1
  Product_7c664/1 -> Divide_9cc5b/1
  Constant_T_w_abd95/1 -> Divide_9cc5b/2
  Add_a5b72/1 -> Divide_96d2f/1
  Constant_T_w_e0452/1 -> Divide_96d2f/2
  Divide_9cc5b/1 -> Add_9667d/1
  Divide_96d2f/1 -> Add_9667d/2
  Constant_T_2_01690/1 -> Product_7477e/1
  Add_9667d/1 -> Product_7477e/2
  State_Px_1_SG_D_2_be7f9/1 -> Add_05d88/1
  Product_7b0e8/1 -> Divide_6c654/1
  Constant_T_1_fc97c/1 -> Divide_6c654/2
  Add_05d88/1 -> Divide_83357/1
  Constant_T_1_b6bc0/1 -> Divide_83357/2
  Divide_6c654/1 -> Add_b38f2/1
  Divide_83357/1 -> Add_b38f2/2
  Add_b38f2/1 -> Blockout_d_Px_2_SG_D_2_a6ada/1

== system IEEE9_case/SG_D_2/d_Px_3_SG_D_2_block ==
  note: d_Px_3_SG_D_2 in IEEE9_case
      | $\frac{\mathrm{Px}_{2,\mathrm{SG},D,2}+T_{4}\,\left(\frac{\mathrm{Px}_{1,\mathrm{SG},D,2}-T_{2}\,\left(\frac{\mathrm{Px}_{1,\mathrm{SG},D,2}}{T_{w}}-\frac{w_{\mathrm{SG},D,2}-2\,\pi \,f_{0}}{T_{w}}\right)}{T_{1}}-\frac{\mathrm{Px}_{2,\mathrm{SG},D,2}}{T_{1}}\right)}{T_{3}}-\frac{\mathrm{Px}_{3,\mathrm{SG},D,2}}{T_{3}}$
      | Automatically generated on 2025-11-01 08:49:17 .
  State_Px_3_SG_D_2_e98da : Inport
  State_Px_2_SG_D_2_44f04 : Inport  Port=2
  State_Px_2_SG_D_2_acc18 : Inport  Port=3
  State_Px_1_SG_D_2_79294 : Inport  Port=4
  State_Px_1_SG_D_2_44be4 : Inport  Port=5
  State_w_SG_D_2_71684 : Inport  Port=6
  Add_58979 : Sum
  Add_69bb2 : Sum
  Add_bd190 : Sum
  Add_be19d : Sum
  Add_d9576 : Sum
  Add_e673d : Sum
  Constant_-1_93d95 : Constant  Value=-1
  Constant_-1_add11 : Constant  Value=-1
  Constant_-1_e53e8 : Constant  Value=-1
  Constant_-2.0_f4fc2 : Constant  Value=-2.0
  Constant_T_1_4b81c : Constant  Value=T_1
  Constant_T_1_873dd : Constant  Value=T_1
  Constant_T_2_fba97 : Constant  Value=T_2
  Constant_T_3_dec50 : Constant  Value=T_3
  Constant_T_3_eced2 : Constant  Value=T_3
  Constant_T_4_37f91 : Constant  Value=T_4
  Constant_T_w_79185 : Constant  Value=T_w
  Constant_T_w_a672d : Constant  Value=T_w
  Constant_f0_e479f : Constant  Value=f0
  Constant_pi_801d6 : Constant  Value=pi
  Divide_0611c : Product  Inputs=*/
  Divide_4876b : Product  Inputs=*/
  Divide_4a63c : Product  Inputs=*/
  Divide_84550 : Product  Inputs=*/
  Divide_84a47 : Product  Inputs=*/
  Divide_e2bfc : Product  Inputs=*/
  Product_0b2e0 : Product
  Product_0cde6 : Product
  Product_24493 : Product
  Product_2c8d8 : Product
  Product_7b0fa : Product
  Product_83b4e : Product
  Product_e1479 : Product
  Blockout_d_Px_3_SG_D_2_2df83 : Outport
  wires:
  Constant_-2.0_f4fc2/1 -> Product_e1479/1
  State_w_SG_D_2_71684/1 -> Add_be19d/2
  Add_e673d/1 -> Divide_84a47/1
  Constant_pi_801d6/1 -> Product_e1479/2
  Constant_-1_add11/1 -> Product_7b0fa/1
  Product_e1479/1 -> Product_2c8d8/1
  State_Px_2_SG_D_2_acc18/1 -> Product_7b0fa/2
  State_Px_1_SG_D_2_44be4/1 -> Product_0b2e0/2
  Divide_84a47/1 -> Add_bd190/2
  Constant_f0_e479f/1 -> Product_2c8d8/2
  Constant_-1_e53e8/1 -> Product_0b2e0/1
  Product_2c8d8/1 -> Add_be19d/1
  Product_0b2e0/1 -> Divide_4a63c/1
  Constant_T_w_a672d/1 -> Divide_4a63c/2
  Divide_0611c/1 -> Add_bd190/1
  Add_be19d/1 -> Divide_84550/1
  Product_24493/1 -> Add_58979/2
  Constant_T_w_79185/1 -> Divide_84550/2
  Divide_4a63c/1 -> Add_69bb2/1
  State_Px_1_SG_D_2_79294/1 -> Add_58979/1
  Divide_84550/1 -> Add_69bb2/2
  Constant_-1_93d95/1 -> Product_83b4e/1
  Constant_T_2_fba97/1 -> Product_24493/1
  Add_69bb2/1 -> Product_24493/2
  Product_7b0fa/1 -> Divide_4876b/1
  Constant_T_1_4b81c/1 -> Divide_4876b/2
  Add_58979/1 -> Divide_e2bfc/1
  Constant_T_1_873dd/1 -> Divide_e2bfc/2
  Divide_4876b/1 -> Add_d9576/1
  Divide_e2bfc/1 -> Add_d9576/2
  Constant_T_4_37f91/1 -> Product_0cde6/1
  Add_d9576/1 -> Product_0cde6/2
  State_Px_3_SG_D_2_e98da/1 -> Product_83b4e/2
  State_Px_2_SG_D_2_44f04/1 -> Add_e673d/1
  Product_0cde6/1 -> Add_e673d/2
  Product_83b4e/1 -> Divide_0611c/1
  Constant_T_3_dec50/1 -> Divide_0611c/2
  Constant_T_3_eced2/1 -> Divide_84a47/2
  Add_bd190/1 -> Blockout_d_Px_3_SG_D_2_2df83/1

== system IEEE9_case/SG_D_2/d_R_f_SG_D_2_block ==
  note: d_R_f_SG_D_2 in IEEE9_case
      | $-\frac{R_{f,\mathrm{SG},D,2}-\frac{E_{\mathrm{fd},\mathrm{SG},D,2}\,K_{F}}{T_{F}}}{T_{F}}$
      | Automatically generated on 2025-11-01 08:49:10 .
  State_E_fd_SG_D_2_c2b5e : Inport
  State_R_f_SG_D_2_17e2e : Inport  Port=2
  Constant_K_F_aee36 : Constant  Value=K_F
  Constant_T_F_f06da : Constant  Value=T_F
  Constant_T_F_f6373 : Constant  Value=T_F
  Divide_5ccae : Product  Inputs=*/
  Divide_df208 : Product  Inputs=*/
  Product_5657b : Product
  Subtract_56e6f : Sum  Inputs=+-
  Blockout_d_R_f_SG_D_2_96516 : Outport
  wires:
  Constant_T_F_f6373/1 -> Divide_df208/2
  State_E_fd_SG_D_2_c2b5e/1 -> Product_5657b/1
  Constant_K_F_aee36/1 -> Product_5657b/2
  State_R_f_SG_D_2_17e2e/1 -> Subtract_56e6f/2
  Product_5657b/1 -> Divide_df208/1
  Divide_df208/1 -> Subtract_56e6f/1
  Constant_T_F_f06da/1 -> Divide_5ccae/2
  Subtract_56e6f/1 -> Divide_5ccae/1
  Divide_5ccae/1 -> Blockout_d_R_f_SG_D_2_96516/1

== system IEEE9_case/SG_D_2/d_T_m_SG_D_2_block ==
  note: d_T_m_SG_D_2 in IEEE9_case
      | $-\frac{T_{m,\mathrm{SG},D,2}-T_{0}+\frac{\mathrm{SpeedPara}\,\left(w_{\mathrm{SG},D,2}-w_{\mathrm{ref}}\right)}{2\,f_{0}\,\pi }}{T_{\mathrm{speed}}}$
      | Automatically generated on 2025-11-01 08:49:01 .
  State_w_SG_D_2_27a0d : Inport
  State_T_m_SG_D_2_c6b35 : Inport  Port=2
  Add_07dc9 : Sum
  Add_27c19 : Sum
  Constant_-1_df1fc : Constant  Value=-1
  Constant_2.0_1a009 : Constant  Value=2.0
  Constant_SpeedPara_3b191 : Constant  Value=SpeedPara
  Constant_T_0_27244 : Constant  Value=T_0
  Constant_T_speed_136b8 : Constant  Value=T_speed
  Constant_f0_4a65e : Constant  Value=f0
  Constant_pi_49b14 : Constant  Value=pi
  Constant_w_ref_0eb21 : Constant  Value=w_ref
  Divide_06317 : Product  Inputs=*/
  Divide_0e6d1 : Product  Inputs=*/
  Product_31695 : Product
  Product_bf0fb : Product
  Product_e86c2 : Product
  Product_f8fb3 : Product
  Subtract_2120d : Sum  Inputs=+-
  Blockout_d_T_m_SG_D_2_0f7e5 : Outport
  wires:
  Constant_pi_49b14/1 -> Product_31695/2
  Constant_-1_df1fc/1 -> Product_bf0fb/1
  Constant_w_ref_0eb21/1 -> Add_27c19/2
  State_w_SG_D_2_27a0d/1 -> Product_bf0fb/2
  Product_bf0fb/1 -> Add_27c19/1
  Add_07dc9/1 -> Subtract_2120d/1
  Add_27c19/1 -> Product_e86c2/2
  Constant_2.0_1a009/1 -> Product_31695/1
  Constant_SpeedPara_3b191/1 -> Product_e86c2/1
  Product_31695/1 -> Product_f8fb3/1
  Constant_f0_4a65e/1 -> Product_f8fb3/2
  Product_e86c2/1 -> Divide_0e6d1/1
  Product_f8fb3/1 -> Divide_0e6d1/2
  Divide_0e6d1/1 -> Add_07dc9/1
  Constant_T_0_27244/1 -> Add_07dc9/2
  State_T_m_SG_D_2_c6b35/1 -> Subtract_2120d/2
  Subtract_2120d/1 -> Divide_06317/1
  Constant_T_speed_136b8/1 -> Divide_06317/2
  Divide_06317/1 -> Blockout_d_T_m_SG_D_2_0f7e5/1

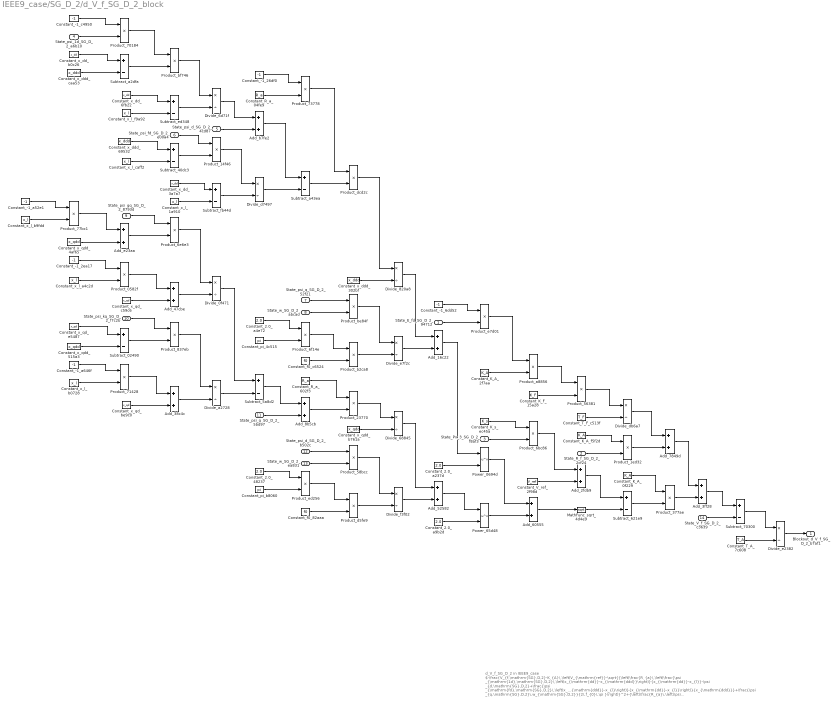
== system IEEE9_case/SG_D_2/d_V_f_SG_D_2_block ==
  note: d_V_f_SG_D_2 in IEEE9_case
      | $-\frac{V_{f,\mathrm{SG},D,2}-K_{A}\,\left(V_{\mathrm{ref}}-\sqrt{{\left(\frac{R_{a}\,\left(\frac{\psi _{\mathrm{1d},\mathrm{SG},D,2}\,\left(x_{\mathrm{dd}}-x_{\mathrm{ddd}}\right)}{x_{\mathrm{dd}}-x_{l}}-\psi _{d,\mathrm{SG},D,2}+\frac{\psi _{\mathrm{fd},\mathrm{SG},D,2}\,\left(x_{\mathrm{ddd}}-x_{l}\right)}{x_{\mathrm{dd}}-x_{l}}\right)}{x_{\mathrm{ddd}}}+\frac{\psi _{q,\mathrm{SG},D,2}\,w_{\mathrm{SG},D,2}}{2\,f_{0}\,\pi }\right)}^2+{\left(\frac{R_{a}\,\left(\psi _{q,\mathrm{SG},D,2}+\frac{\psi _{\mathrm{gq},\mathrm{SG},D,2}\,\left(x_{l}-x_{\mathrm{qdd}}\right)}{x_{l}-x_{\mathrm{qd}}}+\frac{\psi _{\mathrm{kq},\mathrm{SG},D,2}\,\left(x_{\mathrm{qd}}-x_{\mathrm{qdd}}\right)}{x_{l}-x_{\mathrm{qd}}}\right)}{x_{\mathrm{qdd}}}+\frac{\psi _{d,\mathrm{SG},D,2}\,w_{\mathrm{SG},D,2}}{2\,f_{0}\,\pi }\right)}^2}+K_{s}\,\mathrm{Px}_{3,\mathrm{SG},D,2}\right)-K_{A}\,R_{f,\mathrm{SG},D,2}+\frac{E_{\mathrm{fd},\mathrm{SG},D,2}\,K_{A}\,K_{F}}{T_{F}}}{T_{A}}$
      | Automatically generated on 2025-11-01 08:49:08 .
  State_E_fd_SG_D_2_94712 : Inport
  State_R_f_SG_D_2_2cf24 : Inport  Port=2
  State_Px_3_SG_D_2_f8af3 : Inport  Port=3
  State_psi_1d_SG_D_2_a6b10 : Inport  Port=4
  State_psi_d_SG_D_2_4cd87 : Inport  Port=5
  State_psi_fd_SG_D_2_e00a4 : Inport  Port=6
  State_psi_q_SG_D_2_52f21 : Inport  Port=7
  State_w_SG_D_2_abcad : Inport  Port=8
  State_psi_gq_SG_D_2_8793d : Inport  Port=9
  State_psi_kq_SG_D_2_f7c2b : Inport  Port=10
  State_psi_q_SG_D_2_5bd97 : Inport  Port=11
  State_psi_d_SG_D_2_b502c : Inport  Port=12
  State_w_SG_D_2_ea831 : Inport  Port=13
  State_V_f_SG_D_2_c3639 : Inport  Port=14
  Add_16c22 : Sum
  Add_2fdb9 : Sum
  Add_38c4c : Sum
  Add_3ff28 : Sum
  Add_47cbe : Sum
  Add_52582 : Sum
  Add_60555 : Sum
  Add_7849d : Sum
  Add_8b5cb : Sum
  Add_b7fe2 : Sum
  Add_e23aa : Sum
  Constant_-1_26df0 : Constant  Value=-1
  Constant_-1_2ea17 : Constant  Value=-1
  Constant_-1_6dd52 : Constant  Value=-1
  Constant_-1_a52e1 : Constant  Value=-1
  Constant_-1_a646f : Constant  Value=-1
  Constant_-1_c4950 : Constant  Value=-1
  Constant_2.0_48237 : Constant  Value=2.0
  Constant_2.0_a237d : Constant  Value=2.0
  Constant_2.0_a4e72 : Constant  Value=2.0
  Constant_2.0_a9b2d : Constant  Value=2.0
  Constant_K_A_0f229 : Constant  Value=K_A
  Constant_K_A_2f7aa : Constant  Value=K_A
  Constant_K_A_f5f2d : Constant  Value=K_A
  Constant_K_F_15a28 : Constant  Value=K_F
  Constant_K_s_ec45a : Constant  Value=K_s
  Constant_R_a_04fe9 : Constant  Value=R_a
  Constant_R_a_602f3 : Constant  Value=R_a
  Constant_T_A_7c608 : Constant  Value=T_A
  Constant_T_F_c513f : Constant  Value=T_F
  Constant_V_ref_2f98d : Constant  Value=V_ref
  Constant_f0_82aaa : Constant  Value=f0
  Constant_f0_c6524 : Constant  Value=f0
  Constant_pi_4c515 : Constant  Value=pi
  Constant_pi_b8060 : Constant  Value=pi
  Constant_x_dd_3a7a7 : Constant  Value=x_dd
  Constant_x_dd_6fb22 : Constant  Value=x_dd
  Constant_x_dd_b0c26 : Constant  Value=x_dd
  Constant_x_ddd_302bf : Constant  Value=x_ddd
  Constant_x_ddd_69532 : Constant  Value=x_ddd
  Constant_x_ddd_caa53 : Constant  Value=x_ddd
  Constant_x_l_1a910 : Constant  Value=x_l
  Constant_x_l_a4c2d : Constant  Value=x_l
  Constant_x_l_b0728 : Constant  Value=x_l
  Constant_x_l_b9fdd : Constant  Value=x_l
  Constant_x_l_caff2 : Constant  Value=x_l
  Constant_x_l_f9a92 : Constant  Value=x_l
  Constant_x_qd_be9c0 : Constant  Value=x_qd
  Constant_x_qd_c59c6 : Constant  Value=x_qd
  Constant_x_qd_e5487 : Constant  Value=x_qd
  Constant_x_qdd_4af65 : Constant  Value=x_qdd
  Constant_x_qdd_515a3 : Constant  Value=x_qdd
  Constant_x_qdd_b761a : Constant  Value=x_qdd
  Divide_0f471 : Product  Inputs=*/
  Divide_68845 : Product  Inputs=*/
  Divide_6d71f : Product  Inputs=*/
  Divide_820a8 : Product  Inputs=*/
  Divide_a2728 : Product  Inputs=*/
  Divide_d7497 : Product  Inputs=*/
  Divide_db6a7 : Product  Inputs=*/
  Divide_e2382 : Product  Inputs=*/
  Divide_e7f2c : Product  Inputs=*/
  Divide_f3f02 : Product  Inputs=*/
  MathFunc_sqrt_4d4e9 : Sqrt
  Power_0694d : Math  Operator=pow
  Power_65d48 : Math  Operator=pow
  Product_0582f : Product
  Product_14f46 : Product
  Product_1ed32 : Product
  Product_{23770,56381,70184,71428,73778} (5 alike) : Product
  Product_377ae : Product
  Product_58bcc : Product
  Product_6bc86 : Product
  Product_6e6e3 : Product
  Product_6f14e : Product
  Product_77bc1 : Product
  Product_837eb : Product
  Product_a8856 : Product
  Product_b2ca8 : Product
  Product_be84f : Product
  Product_bf746 : Product
  Product_d5fe9 : Product
  Product_dcd2c : Product
  Product_e7d01 : Product
  Product_ed256 : Product
  Subtract_02490 : Sum  Inputs=+-
  Subtract_40dc3 : Sum  Inputs=+-
  Subtract_5a8d2 : Sum  Inputs=+-
  Subtract_621e9 : Sum  Inputs=+-
  Subtract_70300 : Sum  Inputs=+-
  Subtract_a2dfa : Sum  Inputs=+-
  Subtract_a43ea : Sum  Inputs=+-
  Subtract_ed348 : Sum  Inputs=+-
  Subtract_fb44d : Sum  Inputs=+-
  Blockout_d_V_f_SG_D_2_b7af1 : Outport
  wires:
  Constant_-1_c4950/1 -> Product_70184/1
  Constant_2.0_a4e72/1 -> Product_6f14e/1
  Constant_-1_a52e1/1 -> Product_77bc1/1
  Product_6f14e/1 -> Product_b2ca8/1
  Product_77bc1/1 -> Add_e23aa/1
  Constant_x_l_b0728/1 -> Product_71428/2
  Constant_x_l_b9fdd/1 -> Product_77bc1/2
  State_psi_1d_SG_D_2_a6b10/1 -> Product_70184/2
  Constant_x_l_1a910/1 -> Subtract_fb44d/2
  Constant_x_dd_b0c26/1 -> Subtract_a2dfa/1
  Product_23770/1 -> Divide_68845/1
  Constant_x_ddd_caa53/1 -> Subtract_a2dfa/2
  Constant_x_qd_be9c0/1 -> Add_38c4c/2
  Add_e23aa/1 -> Product_6e6e3/2
  Constant_x_qdd_4af65/1 -> Add_e23aa/2
  Constant_-1_2ea17/1 -> Product_0582f/1
  Constant_x_dd_3a7a7/1 -> Subtract_fb44d/1
  Subtract_5a8d2/1 -> Add_8b5cb/1
  Power_0694d/1 -> Add_60555/1
  Constant_x_l_a4c2d/1 -> Product_0582f/2
  Constant_2.0_48237/1 -> Product_ed256/1
  Constant_x_qd_e5487/1 -> Subtract_02490/1
  Constant_pi_b8060/1 -> Product_ed256/2
  Subtract_a43ea/1 -> Product_dcd2c/2
  Constant_x_qdd_515a3/1 -> Subtract_02490/2
  State_psi_fd_SG_D_2_e00a4/1 -> Product_14f46/1
  Constant_-1_a646f/1 -> Product_71428/1
  Product_70184/1 -> Product_bf746/1
  State_w_SG_D_2_ea831/1 -> Product_58bcc/2
  Subtract_a2dfa/1 -> Product_bf746/2
  Constant_x_dd_6fb22/1 -> Subtract_ed348/1
  State_psi_q_SG_D_2_5bd97/1 -> Add_8b5cb/2
  State_w_SG_D_2_abcad/1 -> Product_be84f/2
  Subtract_40dc3/1 -> Product_14f46/2
  Constant_x_l_f9a92/1 -> Subtract_ed348/2
  Add_7849d/1 -> Add_3ff28/1
  Constant_x_ddd_69532/1 -> Subtract_40dc3/1
  Constant_x_l_caff2/1 -> Subtract_40dc3/2
  State_psi_gq_SG_D_2_8793d/1 -> Product_6e6e3/1
  Product_0582f/1 -> Add_47cbe/1
  Subtract_fb44d/1 -> Divide_d7497/2
  Constant_x_qd_c59c6/1 -> Add_47cbe/2
  Product_be84f/1 -> Divide_e7f2c/1
  State_psi_kq_SG_D_2_f7c2b/1 -> Product_837eb/1
  Subtract_02490/1 -> Product_837eb/2
  Product_14f46/1 -> Divide_d7497/1
  State_V_f_SG_D_2_c3639/1 -> Subtract_70300/2
  Product_71428/1 -> Add_38c4c/1
  Product_bf746/1 -> Divide_6d71f/1
  Divide_0f471/1 -> Subtract_5a8d2/1
  Subtract_ed348/1 -> Divide_6d71f/2
  Product_6e6e3/1 -> Divide_0f471/1
  Add_47cbe/1 -> Divide_0f471/2
  Product_837eb/1 -> Divide_a2728/1
  Divide_d7497/1 -> Subtract_a43ea/2
  Constant_f0_c6524/1 -> Product_b2ca8/2
  Add_38c4c/1 -> Divide_a2728/2
  Divide_6d71f/1 -> Add_b7fe2/1
  State_psi_d_SG_D_2_4cd87/1 -> Add_b7fe2/2
  Divide_a2728/1 -> Subtract_5a8d2/2
  Constant_-1_26df0/1 -> Product_73778/1
  Constant_R_a_04fe9/1 -> Product_73778/2
  Constant_f0_82aaa/1 -> Product_d5fe9/2
  Add_b7fe2/1 -> Subtract_a43ea/1
  Product_73778/1 -> Product_dcd2c/1
  Constant_pi_4c515/1 -> Product_6f14e/2
  State_psi_q_SG_D_2_52f21/1 -> Product_be84f/1
  Constant_R_a_602f3/1 -> Product_23770/1
  State_E_fd_SG_D_2_94712/1 -> Product_e7d01/2
  Add_8b5cb/1 -> Product_23770/2
  State_psi_d_SG_D_2_b502c/1 -> Product_58bcc/1
  Product_ed256/1 -> Product_d5fe9/1
  Product_dcd2c/1 -> Divide_820a8/1
  Constant_x_ddd_302bf/1 -> Divide_820a8/2
  Product_b2ca8/1 -> Divide_e7f2c/2
  Constant_x_qdd_b761a/1 -> Divide_68845/2
  Product_58bcc/1 -> Divide_f3f02/1
  Product_d5fe9/1 -> Divide_f3f02/2
  Divide_820a8/1 -> Add_16c22/1
  Divide_e7f2c/1 -> Add_16c22/2
  Divide_68845/1 -> Add_52582/1
  Divide_f3f02/1 -> Add_52582/2
  Constant_-1_6dd52/1 -> Product_e7d01/1
  Add_16c22/1 -> Power_0694d/1
  Constant_2.0_a237d/1 -> Power_0694d/2
  Add_52582/1 -> Power_65d48/1
  Constant_2.0_a9b2d/1 -> Power_65d48/2
  Product_e7d01/1 -> Product_a8856/1
  Constant_K_A_2f7aa/1 -> Product_a8856/2
  Constant_K_s_ec45a/1 -> Product_6bc86/1
  State_Px_3_SG_D_2_f8af3/1 -> Product_6bc86/2
  Power_65d48/1 -> Add_60555/2
  Product_a8856/1 -> Product_56381/1
  Constant_K_F_15a28/1 -> Product_56381/2
  Product_6bc86/1 -> Add_2fdb9/1
  Constant_V_ref_2f98d/1 -> Add_2fdb9/2
  Add_60555/1 -> MathFunc_sqrt_4d4e9/1
  Product_56381/1 -> Divide_db6a7/1
  Constant_T_F_c513f/1 -> Divide_db6a7/2
  Constant_K_A_f5f2d/1 -> Product_1ed32/1
  State_R_f_SG_D_2_2cf24/1 -> Product_1ed32/2
  Add_2fdb9/1 -> Subtract_621e9/1
  MathFunc_sqrt_4d4e9/1 -> Subtract_621e9/2
  Divide_db6a7/1 -> Add_7849d/1
  Product_1ed32/1 -> Add_7849d/2
  Constant_K_A_0f229/1 -> Product_377ae/1
  Subtract_621e9/1 -> Product_377ae/2
  Product_377ae/1 -> Add_3ff28/2
  Add_3ff28/1 -> Subtract_70300/1
  Subtract_70300/1 -> Divide_e2382/1
  Constant_T_A_7c608/1 -> Divide_e2382/2
  Divide_e2382/1 -> Blockout_d_V_f_SG_D_2_b7af1/1
